simulink model "ec_fixed_slm_with_bypass_reset"  (Simulink 10.0)
settings: Solver=FixedStepDiscrete  StartTime=0.0  StopTime=20  RelTol=1e-3
PreLoadFcn:
  | ec_fixed_setup;
StartFcn:
  | tic;
StopFcn:
  | toc;
undefined symbols (not defined in the file): ec_length, Fs, pic_frame_size, sm_length, spkr_to_mic_delay, spkr_to_mic_filter
libraries: dspsnks4 x5, dspsrcs4 x4, simulink x2, commchan3 x2, dspmathops x2, dspsigops x1, dspadpt3 x1, dspmtrx3 x1, ec_lib x1
settings Model: Creator=Kerry Schutz  LastModifiedBy=bhisma
settings DataIOCC: LimitDataPoints=on  SignalLoggingSaveFormat=ModelDataLogs
settings OptimizationCC: DefaultParameterBehavior=Inlined  InlineInvariantSignals=on  ExpressionDepthLimit=2147483647  StateBitsets=on  DataBitsets=on  ZeroExternalMemoryAtStartup=off  ZeroInternalMemoryAtStartup=off  EfficientFloat2IntCast=on  LifeSpan=1  EfficientTunableParamExpr=on
settings DebuggingCC: AlgebraicLoopMsg=none  SaveWithParameterizedLinksMsg=none  SolverPrmCheckMsg=warning  FcnCallInpInsideContextMsg=warning  StateNameClashWarn=warning
settings HardwareCC: ProdBitPerInt=16  ProdBitPerPointer=16  ProdBitPerSizeT=16  ProdBitPerPtrDiffT=16  ProdIntDivRoundTo=Zero  ProdEndianess=LittleEndian  ProdWordSize=16  ProdHWDeviceType=Microchip->dsPIC  TargetHWDeviceType=32-bit Generic
settings SFSimCC: SimUseLocalCustomCode=on  SimParseCustomCode=off  MATLABDynamicMemAlloc=off  CustomCodeUndefinedFunction=FilterOut
settings RTWCC: Description=Real-Time Workshop Embedded Coder (no auto configuration)  SystemTargetFile=ert.tlc  GenCodeOnly=on  TemplateMakefile=ert_default_tmf  RTWUseLocalCustomCode=on  CreateSILPILBlock=SIL
settings CodeAppCC: IgnoreCustomStorageClasses=off  CustomSymbolStrType=$N$R$M  InternalIdentifier=Classic  InlinedPrmAccess=Macros
settings ERTTargetCC: TargetFcnLib=ansi_tfl_tmw.mat  GenerateSampleERTMain=on  IncludeMdlTerminateFcn=off  SupportAbsoluteTime=off  PurelyIntegerCode=on  SupportNonFinite=off  SupportComplex=off  InlinedParameterPlacement=NonHierarchical  ERTCustomFileTemplate=example_file_process.tlc  ConvertIfToSwitch=off  SuppressUnreachableDefaultCases=off

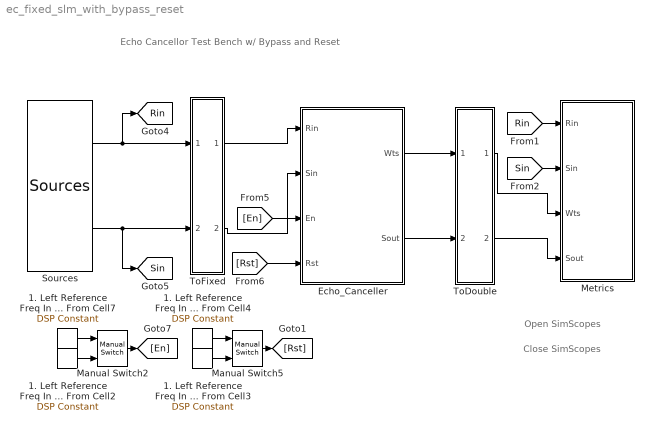
== system ec_fixed_slm_with_bypass_reset ==
  note: Echo Cancellor Test Bench w/ Bypass and Reset
  note: Close SimScopes
  note: Open SimScopes
  1. Left Reference Freq In Hz From Cell2 : dspsrcs4/DSP Constant  SystemSampleTime=-1  Value=0  SampleMode=Discrete  discreteOutput=Sample-based  continuousOutput=Sample-based  sampTime=pic_frame_size/Fs  framePeriod=pic_frame_size/Fs  dataType=int16  isSigned=on  wordLen=16  udDataType=sfix(16)  fracBitsMode=Best precision  numFracBits=15  InterpretAs1D=-inf  Ts=-inf  FramebasedOutput=-inf
      settings: SourceProductName=DSP System Toolbox  SourceProductBaseCode=DS  additionalParams=on
  1. Left Reference Freq In Hz From Cell3 : dspsrcs4/DSP Constant  SystemSampleTime=-1  Value=0  SampleMode=Discrete  discreteOutput=Sample-based  continuousOutput=Sample-based  sampTime=pic_frame_size/Fs  framePeriod=pic_frame_size/Fs  dataType=int16  isSigned=on  wordLen=16  udDataType=sfix(16)  fracBitsMode=Best precision  numFracBits=15  InterpretAs1D=-inf  Ts=-inf  FramebasedOutput=-inf
      settings: SourceProductName=DSP System Toolbox  SourceProductBaseCode=DS  additionalParams=on
  1. Left Reference Freq In Hz From Cell4 : dspsrcs4/DSP Constant  SystemSampleTime=-1  Value=1  SampleMode=Discrete  discreteOutput=Sample-based  continuousOutput=Sample-based  sampTime=pic_frame_size/Fs  framePeriod=pic_frame_size/Fs  dataType=int16  isSigned=on  wordLen=16  udDataType=sfix(16)  fracBitsMode=Best precision  numFracBits=15  InterpretAs1D=-inf  Ts=-inf  FramebasedOutput=-inf
      settings: SourceProductName=DSP System Toolbox  SourceProductBaseCode=DS  additionalParams=on
  1. Left Reference Freq In Hz From Cell7 : dspsrcs4/DSP Constant  SystemSampleTime=-1  Value=1  SampleMode=Discrete  discreteOutput=Sample-based  continuousOutput=Sample-based  sampTime=pic_frame_size/Fs  framePeriod=pic_frame_size/Fs  dataType=int16  isSigned=on  wordLen=16  udDataType=sfix(16)  fracBitsMode=Best precision  numFracBits=15  InterpretAs1D=-inf  Ts=-inf  FramebasedOutput=-inf
      settings: SourceProductName=DSP System Toolbox  SourceProductBaseCode=DS  additionalParams=on
  Echo_Canceller : Subsystem
  Manual Switch2 : simulink/Signal Routing/Manual Switch  SystemSampleTime=-1  sw=1  action=0  varsize=off
      settings: SourceProductName=Simulink  SourceProductBaseCode=SL
  Manual Switch5 : simulink/Signal Routing/Manual Switch  SystemSampleTime=-1  sw=0  action=0  varsize=off
      settings: SourceProductName=Simulink  SourceProductBaseCode=SL
  Metrics : Subsystem  TreatAsAtomicUnit=on
  Sources : ec_lib/Sources  SystemSampleTime=-1
  ToDouble : Subsystem
  ToFixed : Subsystem
  tag scope: Rin=global, Sin=global
  wires:
  ToFixed/1(Rin) -> Echo_Canceller/1(Rin)
  ToFixed/2(Sin) -> Echo_Canceller/2("Sin ")
  Echo_Canceller/1(Wts) -> ToDouble/1(In1)
  Echo_Canceller/2(Sout) -> ToDouble/2(In2)
  Sources/2 -> ToFixed/2(" In2"), [Sin]
  Sources/1 -> ToFixed/1(In1), [Rin]
  ToDouble/1(Wts) -> Metrics/3(Wts)
  ToDouble/2(Sout) -> Metrics/4(Sout)
  [Rin] -> Metrics/1(Rin)
  [Sin] -> Metrics/2(Sin)
  1. Left Reference Freq In Hz From Cell7/1 -> Manual Switch2/1
  Manual Switch2/1 -> [En]
  1. Left Reference Freq In Hz From Cell2/1 -> Manual Switch2/2
  [En] -> Echo_Canceller/3(En)
  [Rst] -> Echo_Canceller/4(Rst)
  1. Left Reference Freq In Hz From Cell4/1 -> Manual Switch5/1
  Manual Switch5/1 -> [Rst]
  1. Left Reference Freq In Hz From Cell3/1 -> Manual Switch5/2

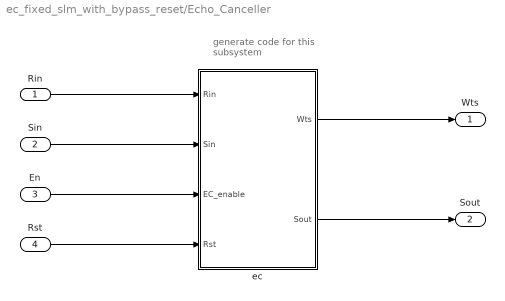
== system ec_fixed_slm_with_bypass_reset/Echo_Canceller ==
  note: generate code for this
      | subsystem
  Rin : Inport
  "Sin " : Inport  Port=2
  En : Inport  Port=3  OutDataTypeStr=int16
  Rst : Inport  Port=4  OutDataTypeStr=int16
  ec : Subsystem
  Wts : Outport
  Sout : Outport  Port=2
  wires:
  Rin/1 -> ec/1(Rin)
  "Sin "/1 -> ec/2(Sin)
  ec/1(Wts) -> Wts/1
  ec/2(Sout) -> Sout/1
  En/1 -> ec/3(EC_enable)
  Rst/1 -> ec/4(Rst)

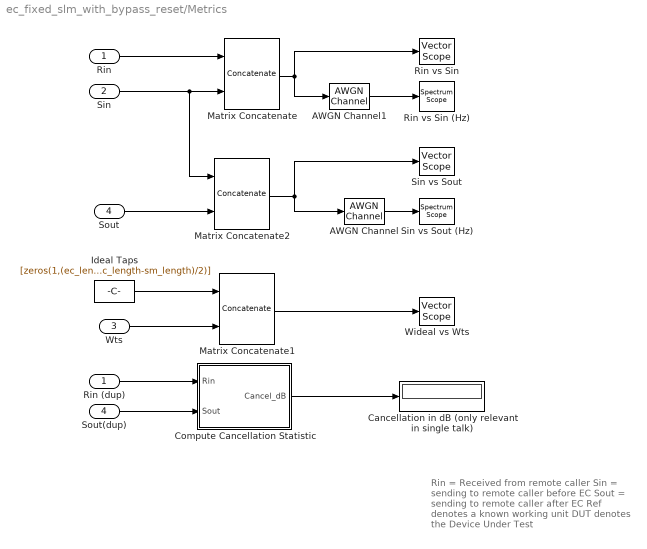
== system ec_fixed_slm_with_bypass_reset/Metrics ==
  note: Rin = Received from remote caller
      | Sin = sending to remote caller before EC
      | Sout = sending to remote caller after EC
      | Ref denotes a known working unit
      | DUT denotes the Device Under Test
  Rin : Inport
  Sin : Inport  Port=2
  Wts : Inport  Port=3
  Sout : Inport  Port=4
  AWGN Channel : commchan3/AWGN Channel  SystemSampleTime=-1  seed=67  noiseMode="Signal to noise ratio  (Eb/No)"  EbNodB=100  EsNodB=10  SNRdB=10  bitsPerSym=1  Ps=1  Tsym=1/Fs  variance=1
      settings: SourceProductName=Communications Toolbox
  AWGN Channel1 : commchan3/AWGN Channel  SystemSampleTime=-1  seed=67  noiseMode="Signal to noise ratio  (Eb/No)"  EbNodB=100  EsNodB=10  SNRdB=10  bitsPerSym=1  Ps=1  Tsym=1/Fs  variance=1
      settings: SourceProductName=Communications Toolbox
  Cancellation in dB (only relevant in single talk) : Display
  Compute Cancellation Statistic : Subsystem
  Ideal Taps : Constant  Value=[zeros(1,(ec_length-sm_length)/2) spkr_to_mic_filter zeros(1,(ec_length-sm_length)/2)]  SampleTime=pic_frame_size/Fs  FramePeriod=pic_frame_size/Fs
      settings: SamplingMode=Frame based
  Matrix Concatenate : Concatenate  Mode=Multidimensional array  ConcatenateDimension=2
  Matrix Concatenate1 : Concatenate  Mode=Multidimensional array  ConcatenateDimension=2
  Matrix Concatenate2 : Concatenate  Mode=Multidimensional array  ConcatenateDimension=2
  Rin (dup) : InportShadow
  Rin vs Sin : dspsnks4/Vector Scope  ScopeProperties=on  Domain=Time  HorizSpan=1  DisplayProperties=off  AxisGrid=on  Memory=off  FrameNumber=on  AxisLegend=off  AxisZoom=off  OpenScopeAtSimStart=off  OpenScopeImmediately=off  FigPos=[21 752 277 182]  AxisProperties=off  XUnits=Hertz  XRange=[0...Fs/2]  InheritXIncr=on  XIncr=1  XLabel=Time  XLimit=Auto  XMin=0  XMax=1  XStart=0  YUnits=dB  YLabel=Amplitude  LineProperties=off  LineColors=[1 0 0]|[0 1 0]
      settings: SourceProductName=DSP System Toolbox  SourceProductBaseCode=DS  YMin=-1  YMax=1
  Rin vs Sin (Hz) : dspsnks4/Spectrum Scope  SystemSampleTime=-1  ScopeProperties=on  Domain=Frequency  HorizSpan=1  UseBuffer=on  BufferSize=512  Overlap=64  inpFftLenInherit=off  FFTlength=128  numAvg=2  DisplayProperties=off  AxisGrid=on  Memory=off  FrameNumber=on  AxisLegend=off  AxisZoom=off  OpenScopeAtSimStart=off  OpenScopeImmediately=off  FigPos=[22 519 280 178]  AxisProperties=off  XUnits=Hertz  XRange=[0...Fs/2]  InheritXIncr=on  XIncr=1.0  XLabel=Samples  XLimit=Auto  YUnits=dB  XMax=1  XMin=0  YLabel=Magnitude-squared, dB  LineProperties=off  LineColors=[1 0 0]|[0 1 0]  wintypeSpecScope=Hann  RsSpecScope=50  betaSpecScope=5  winsampSpecScope=Periodic
      settings: SourceProductName=DSP System Toolbox  SourceProductBaseCode=DS  YMin=-87.2863320440191  YMax=22.6100164436924
  Sin vs Sout : dspsnks4/Vector Scope  ScopeProperties=on  Domain=Time  HorizSpan=1  DisplayProperties=off  AxisGrid=on  Memory=off  FrameNumber=on  AxisLegend=off  AxisZoom=off  OpenScopeAtSimStart=off  OpenScopeImmediately=off  FigPos=[309 518 291 181]  AxisProperties=off  XUnits=Hertz  XRange=[0...Fs/2]  InheritXIncr=on  XIncr=1  XLabel=Time  XLimit=Auto  XMin=0  XMax=1  XStart=0  YUnits=dB  YLabel=Amplitude  LineProperties=off  LineColors=[1 0 0]|[0 1 0]
      settings: SourceProductName=DSP System Toolbox  SourceProductBaseCode=DS  YMin=-1.10854137455551  YMax=1.10983865900285
  Sin vs Sout (Hz) : dspsnks4/Spectrum Scope  SystemSampleTime=-1  ScopeProperties=on  Domain=Frequency  HorizSpan=1  UseBuffer=on  BufferSize=512  Overlap=64  inpFftLenInherit=off  FFTlength=128  numAvg=2  DisplayProperties=off  AxisGrid=on  Memory=off  FrameNumber=on  AxisLegend=off  AxisZoom=off  OpenScopeAtSimStart=off  OpenScopeImmediately=off  FigPos=[313 280 293 181]  AxisProperties=off  XUnits=Hertz  XRange=[0...Fs/2]  InheritXIncr=on  XIncr=1.0  XLabel=Samples  XLimit=Auto  YUnits=dB  XMax=1  XMin=0  YLabel=Magnitude-squared, dB  LineProperties=off  LineColors=[1 0 0]|[0 1 0]  wintypeSpecScope=Hann  RsSpecScope=50  betaSpecScope=5  winsampSpecScope=Periodic
      settings: SourceProductName=DSP System Toolbox  SourceProductBaseCode=DS  YMin=-128.562839071617  YMax=21.0948472865104
  Sout(dup) : InportShadow  Port=4
  Wideal vs Wts : dspsnks4/Vector Scope  ScopeProperties=on  Domain=Time  HorizSpan=1  DisplayProperties=off  AxisGrid=on  Memory=off  FrameNumber=on  AxisLegend=off  AxisZoom=off  OpenScopeAtSimStart=on  OpenScopeImmediately=off  FigPos=[16 440 466 179]  AxisProperties=off  XUnits=Hertz  XRange=[0...Fs/2]  InheritXIncr=on  XIncr=1  XLabel=Time  XLimit=Auto  XMin=0  XMax=1  XStart=0  YUnits=dB  YLabel=Amplitude  LineProperties=off  LineColors=[1 0 0]|[0 1 0]
      settings: SourceProductName=DSP System Toolbox  SourceProductBaseCode=DS  YMin=-0.387806694375187  YMax=0.388477789695183
  wires:
  Sout(dup)/1 -> Compute Cancellation Statistic/2(Sout)
  Rin (dup)/1 -> Compute Cancellation Statistic/1(Rin)
  Sin/1 -> Matrix Concatenate2/1, Matrix Concatenate/2
  Rin/1 -> Matrix Concatenate/1
  Matrix Concatenate/1 -> AWGN Channel1/1, Rin vs Sin/1
  AWGN Channel/1 -> Sin vs Sout (Hz)/1
  AWGN Channel1/1 -> Rin vs Sin (Hz)/1
  Matrix Concatenate1/1 -> Wideal vs Wts/1
  Matrix Concatenate2/1 -> AWGN Channel/1, Sin vs Sout/1
  Ideal Taps/1 -> Matrix Concatenate1/1
  Wts/1 -> Matrix Concatenate1/2
  Sout/1 -> Matrix Concatenate2/2
  Compute Cancellation Statistic/1(Cancel_dB) -> Cancellation in dB (only relevant in single talk)/1

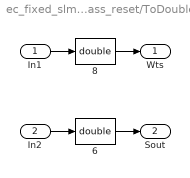
== system ec_fixed_slm_with_bypass_reset/ToDouble ==
  In1 : Inport
  In2 : Inport  Port=2
  " 6" : DataTypeConversion  OutDataTypeStr=double
  " 8" : DataTypeConversion  OutDataTypeStr=double
  Wts : Outport
  Sout : Outport  Port=2
  wires:
  In1/1 -> " 8"/1
  " 8"/1 -> Wts/1
  In2/1 -> " 6"/1
  " 6"/1 -> Sout/1

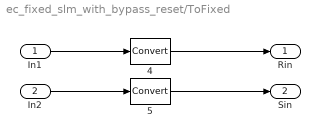
== system ec_fixed_slm_with_bypass_reset/ToFixed ==
  In1 : Inport
  " In2" : Inport  Port=2
  " 4" : DataTypeConversion
  " 5" : DataTypeConversion
  Rin : Outport
  Sin : Outport  Port=2
  wires:
  In1/1 -> " 4"/1
  " 4"/1 -> Rin/1
  " In2"/1 -> " 5"/1
  " 5"/1 -> Sin/1

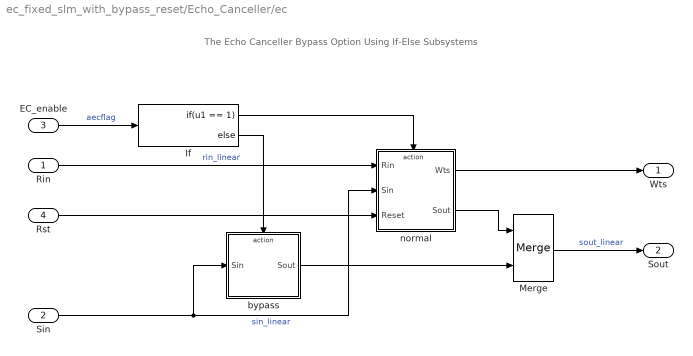
== system ec_fixed_slm_with_bypass_reset/Echo_Canceller/ec ==
  note: The Echo Canceller Bypass Option
      | Using If-Else Subsystems
  Rin : Inport
  Sin : Inport  Port=2
  EC_enable : Inport  Port=3
  Rst : Inport  Port=4
  If : If  IfExpression=u1 == 1
  Merge : Merge
  bypass : Subsystem  TreatAsAtomicUnit=on
  normal : Subsystem  TreatAsAtomicUnit=on
  Wts : Outport
  Sout : Outport  Port=2
  wires:
  Merge/1 -> Sout/1  "sout_linear"
  EC_enable/1 -> If/1  "aecflag"
  If/1 -> normal/Action
  Sin/1 -> normal/2(Sin), bypass/1("Sin ")  "sin_linear"
  Rin/1 -> normal/1(Rin)  "rin_linear"
  If/2 -> bypass/Action
  bypass/1(Sout) -> Merge/2
  normal/1(Wts) -> Wts/1
  normal/2(Sout) -> Merge/1
  Rst/1 -> normal/3(Reset)

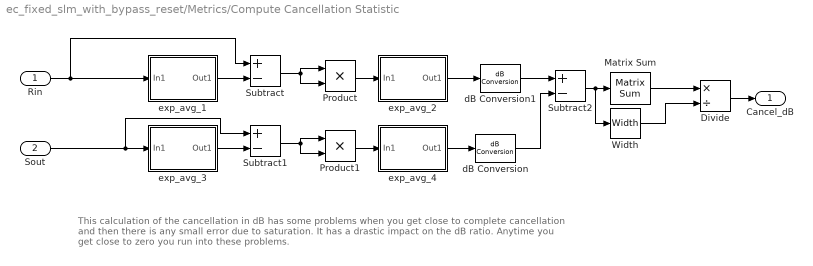
== system ec_fixed_slm_with_bypass_reset/Metrics/Compute Cancellation Statistic ==
  note: This calculation of the cancellation in dB has some problems when you get close to complete cancellation and then there is
      | any small error due to saturation. It has a drastic impact on the dB ratio. Anytime you get close to zero you run into these problems.
  Rin : Inport
  Sout : Inport  Port=2
  Divide : Product  Inputs=*/
  Matrix Sum : dspmtrx3/Matrix Sum  Dim=Columns  outputMode=Binary point scaling  outputWordLength=32  outputFracLength=0  accumMode=Binary point scaling  accumWordLength=32  accumFracLength=0  roundingMode=Floor  overflowMode=off
      settings: SourceProductName=DSP System Toolbox  SourceProductBaseCode=DS  additionalParams=on
  Product : Product  RndMeth=Zero
  Product1 : Product  RndMeth=Zero
  Subtract : Sum  Inputs=+-
  Subtract1 : Sum  Inputs=+-
  Subtract2 : Sum  Inputs=+-
  Width : Width
  dB Conversion : dspmathops/dB Conversion  SystemSampleTime=-1  dBtype=dB  intype=Power  R=1  fuzz=on
      settings: SourceProductName=DSP System Toolbox
  dB Conversion1 : dspmathops/dB Conversion  SystemSampleTime=-1  dBtype=dB  intype=Power  R=1  fuzz=on
      settings: SourceProductName=DSP System Toolbox
  exp_avg_1 : Subsystem
  exp_avg_2 : Subsystem
  exp_avg_3 : Subsystem
  exp_avg_4 : Subsystem
  Cancel_dB : Outport
  wires:
  Rin/1 -> exp_avg_1/1(In1), Subtract/1
  Subtract/1 -> Product/1, Product/2
  Product/1 -> exp_avg_2/1(In1)
  exp_avg_1/1(Out1) -> Subtract/2
  Subtract1/1 -> Product1/2, Product1/1
  Product1/1 -> exp_avg_4/1(In1)
  exp_avg_3/1(Out1) -> Subtract1/2
  dB Conversion/1 -> Subtract2/2
  dB Conversion1/1 -> Subtract2/1
  exp_avg_4/1(Out1) -> dB Conversion/1
  exp_avg_2/1(Out1) -> dB Conversion1/1
  Subtract2/1 -> Width/1, Matrix Sum/1
  Matrix Sum/1 -> Divide/1
  Width/1 -> Divide/2
  Divide/1 -> Cancel_dB/1
  Sout/1 -> exp_avg_3/1(In1), Subtract1/1

== system ec_fixed_slm_with_bypass_reset/Echo_Canceller/ec/bypass ==
  "Sin " : Inport
  Action Port : ActionPort  ActionPortLabel=else { }
  Sout : Outport
  wires:
  "Sin "/1 -> Sout/1

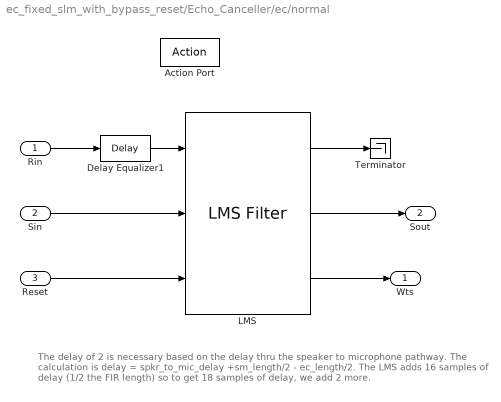
== system ec_fixed_slm_with_bypass_reset/Echo_Canceller/ec/normal ==
  note: The delay of 2 is necessary based on the delay thru the speaker to microphone pathway.
      | The calculation is delay = spkr_to_mic_delay +sm_length/2 - ec_length/2. The LMS
      | adds 16 samples of delay (1/2 the FIR length) so to get 18 samples of delay, we add 2 more.
  Rin : Inport
  Sin : Inport  Port=2
  Reset : Inport  Port=3
  Action Port : ActionPort  ActionPortLabel=if { }
  Delay Equalizer1 : dspsigops/Delay  dly_unit=Samples  delay=spkr_to_mic_delay +sm_length/2 - ec_length/2  ic_detail=off  dif_ic_for_ch=off  dif_ic_for_dly=off  ic=0  reset_popup=None
      settings: SourceProductName=DSP System Toolbox  SourceProductBaseCode=DS
  LMS : dspadpt3/LMS Filter  Algo=LMS  L=ec_length  stepflag=Dialog  mu=300/32768  leakage=1  ic=0  Adapt=off  resetflag=Non-zero sample  weights=on  secondCoeffMode=User-defined  secondCoeffWordLength=2  secondCoeffFracLength=14  accumMode=Binary point scaling  accumWordLength=LMS_Accum_WordLen  accumFracLength=20  accum2Mode=User-defined  accum2FracLength=LMS_Accum_FracLen  prodOutputMode=Binary point scaling  prodOutputWordLength=LMS_Prod_WordLen  prodOutputFracLength=20  prodOutput2Mode=User-defined  prodOutput2FracLength=LMS_Prod_FracLen  prodOutput3Mode=User-defined  prodOutput3FracLength=LMS_Prod_FracLen  prodOutput4Mode=User-defined  prodOutput4FracLength=LMS_Prod_FracLen  quotientMode=User-defined  quotientFracLength=20  memoryMode=Binary point scaling  memoryWordLength=LMS_Wts_WordLen  memoryFracLength=LMS_Wts_FracLen  roundingMode=Nearest  overflowMode=off  addnparflag=off
      settings: SourceProductName=DSP System Toolbox  SourceProductBaseCode=DS
  Terminator : Terminator
  Wts : Outport
  Sout : Outport  Port=2
  wires:
  Rin/1 -> Delay Equalizer1/1
  Sin/1 -> LMS/2
  LMS/1 -> Terminator/1
  LMS/2 -> Sout/1
  LMS/3 -> Wts/1
  Delay Equalizer1/1 -> LMS/1
  Reset/1 -> LMS/3

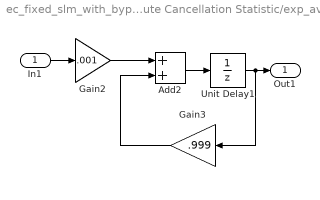
== system ec_fixed_slm_with_bypass_reset/Metrics/Compute Cancellation Statistic/exp_avg_1 ==
  In1 : Inport
  Add2 : Sum
  Gain2 : Gain  Gain=.001
  Gain3 : Gain  Gain=.999
  Unit Delay1 : UnitDelay  SampleTime=-1
  Out1 : Outport
  wires:
  Unit Delay1/1 -> Gain3/1, Out1/1
  In1/1 -> Gain2/1
  Gain3/1 -> Add2/2
  Gain2/1 -> Add2/1
  Add2/1 -> Unit Delay1/1

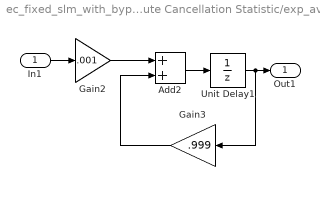
== system ec_fixed_slm_with_bypass_reset/Metrics/Compute Cancellation Statistic/exp_avg_2 ==
  In1 : Inport
  Add2 : Sum
  Gain2 : Gain  Gain=.001
  Gain3 : Gain  Gain=.999
  Unit Delay1 : UnitDelay  SampleTime=-1
  Out1 : Outport
  wires:
  Add2/1 -> Unit Delay1/1
  Gain2/1 -> Add2/1
  Gain3/1 -> Add2/2
  In1/1 -> Gain2/1
  Unit Delay1/1 -> Out1/1, Gain3/1

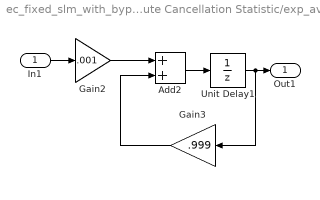
== system ec_fixed_slm_with_bypass_reset/Metrics/Compute Cancellation Statistic/exp_avg_3 ==
  In1 : Inport
  Add2 : Sum
  Gain2 : Gain  Gain=.001
  Gain3 : Gain  Gain=.999
  Unit Delay1 : UnitDelay  SampleTime=-1
  Out1 : Outport
  wires:
  Add2/1 -> Unit Delay1/1
  Gain2/1 -> Add2/1
  Gain3/1 -> Add2/2
  In1/1 -> Gain2/1
  Unit Delay1/1 -> Out1/1, Gain3/1

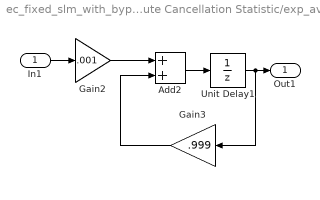
== system ec_fixed_slm_with_bypass_reset/Metrics/Compute Cancellation Statistic/exp_avg_4 ==
  In1 : Inport
  Add2 : Sum
  Gain2 : Gain  Gain=.001
  Gain3 : Gain  Gain=.999
  Unit Delay1 : UnitDelay  SampleTime=-1
  Out1 : Outport
  wires:
  Unit Delay1/1 -> Gain3/1, Out1/1
  In1/1 -> Gain2/1
  Gain3/1 -> Add2/2
  Gain2/1 -> Add2/1
  Add2/1 -> Unit Delay1/1
